simulink model "Complete_System_RatedVoltage"  (R2022b)
settings: Solver=VariableStepAuto  StartTime=0.0  StopTime=10  RelTol=1e-3
model workspace (MAT data in the model file):
  V_3phase = 121
libraries: spsDiodeLib x7, spsACVoltageSourceLib x3, spsMeanLib x2, spsSeriesRLCBranchLib x2, spsCurrentMeasurementLib x1, spsDCMachineLib x1, spsDCVoltageSourceLib x1, spsMosfetLib x1, spsVoltageMeasurementLib x1, spsPWMGeneratorDCDCLib x1, spsVariableRatioTransformerLib x1, sps_lib x1
settings Model: Creator=omers  LastModifiedBy=omers

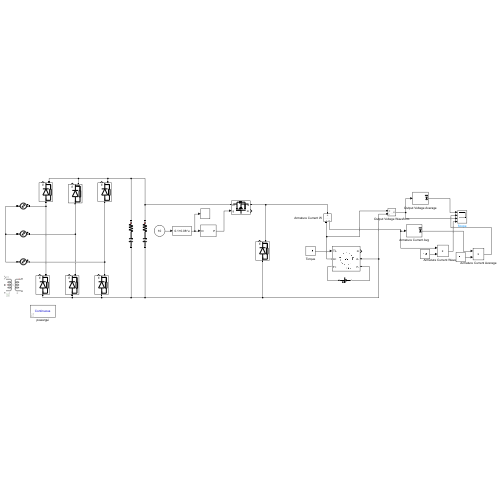
[thumbnail: Simulink's stored preview of the top-level diagram]
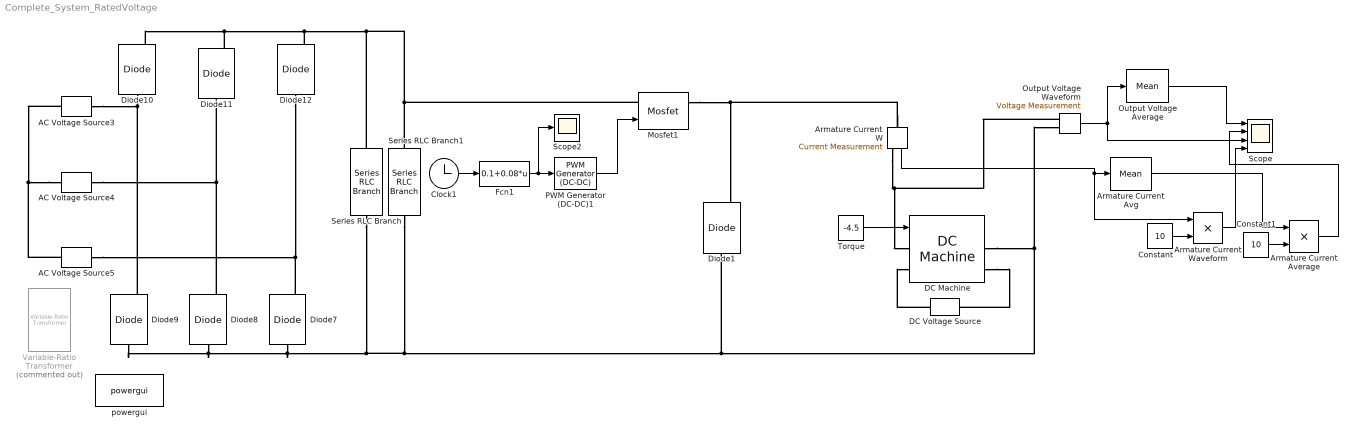
== system Complete_System_RatedVoltage ==
  AC Voltage Source3 : spsACVoltageSourceLib/AC Voltage Source  Amplitude=121  Phase=0  Frequency=50  SampleTime=0  Measurements=None  BusType=swing  Pref=10e3  Qref=0  Qmin=-inf  Qmax=+inf
  AC Voltage Source4 : spsACVoltageSourceLib/AC Voltage Source  Amplitude=121  Phase=-120  Frequency=50  SampleTime=0  Measurements=None  BusType=swing  Pref=10e3  Qref=0  Qmin=-inf  Qmax=+inf
  AC Voltage Source5 : spsACVoltageSourceLib/AC Voltage Source  Amplitude=121  Phase=-240  Frequency=50  SampleTime=0  Measurements=None  BusType=swing  Pref=10e3  Qref=0  Qmin=-inf  Qmax=+inf
  Armature Current Average : Product
  Armature Current Avg : spsMeanLib/Mean  Freq=50  Vinit=0  Ts=0
  Armature Current W : spsCurrentMeasurementLib/Current Measurement  PhasorSimulation=off  OutputType=Complex  PSBequivalent=0
  Armature Current Waveform : Product
  Clock1 : Clock
  Constant : Constant  Value=10
  Constant1 : Constant  Value=10
  DC Machine : spsDCMachineLib/DC Machine  PresetModel=No  MechanicalLoad=Torque TL  FieldType=Wound  ShowDetailedParameters=on  MeasurementBus=off  RLa="[ 0.8  0.0125]"  RLf="[ 210  23]"  Laf=1.8  MachineConstant=Torque constant (N.m/A)  Ke=1.8  Kt=1.8  J=1  Bm=0  Tf=0  w0=1  Ifinit=1.04761904756944  TsPowergui=0  TsBlock=-1
  DC Voltage Source : spsDCVoltageSourceLib/DC Voltage Source  Amplitude=220  Measurements=None
  Diode{1,7..12} (7 alike) : spsDiodeLib/Diode  Ron=0.001  Lon=0  Vf=0.8  IC=0  UseSnubber=0  Rs=500  Cs=250e-9  Measurements=on
  Fcn1 : Fcn  Expr=0.1+0.08*u
  Mosfet1 : spsMosfetLib/Mosfet  Ron=0.1  Lon=0  Rd=0.01  Vfd=0  IC=0  Rs=1e5  Cs=inf  Measurements=on
  Output Voltage Average : spsMeanLib/Mean  Freq=50  Vinit=0  Ts=0
  Output Voltage Waveform : spsVoltageMeasurementLib/Voltage Measurement  PhasorSimulation=off  OutputType=Complex  PSBequivalent=0
  PWM Generator (DC-DC)1 : spsPWMGeneratorDCDCLib/PWM Generator (DC-DC)  Fsw=1000  Ts=0
  Scope : Scope  NumInputPorts=4
  Scope2 : Scope
  Series RLC Branch : spsSeriesRLCBranchLib/Series RLC Branch  LConnTagsString=__new0  RConnTagsString=__new0  BranchType=RC  Resistance=0.0001  Inductance=1e-3  SetiL0=off  InitialCurrent=0  Capacitance=470e-6  Setx0=off  InitialVoltage=0  Measurements=None
  Series RLC Branch1 : spsSeriesRLCBranchLib/Series RLC Branch  LConnTagsString=__new0  RConnTagsString=__new0  BranchType=RC  Resistance=0.0001  Inductance=1e-3  SetiL0=off  InitialCurrent=0  Capacitance=470e-6  Setx0=off  InitialVoltage=0  Measurements=None
  Torque : Constant  Value=-4.5
  Variable-Ratio Transformer : spsVariableRatioTransformerLib/Variable-Ratio Transformer  Commented=on
      settings: LibrarySourceBlock=|
      | sps_lib/Passives/Variable-Ratio
      | Transformer
  powergui : sps_lib/powergui  Priority=1  SimulationMode=Continuous  SampleTime=50e-6  frequency=60  Iterations=50  frequencyindice=0  Pbase=100e6  ErrMax=1e-4  UnitsV=kV  UnitsW=MW  buscounter=0  FunctionMessages=off  echomessages=off  EnableUseOfTLC=off  CurrentSourceSwitches=off  DisableSnubberDevices=off  DisableRonSwitches=off  DisableVfSwitches=off  DisplayEquations=off  AutomaticDiscreteSolvers=off  SolverType=Tustin/Backward Euler (TBE)  Interpol=off  ExternalGateDelay=off  methode=off  Ts=100  x0status=blocks  SPID=on  SwTol=0  HookPort=off  NonlinearTolerance=1e-4  nMaxIteration=100  ContinueOnMaxIteration=off  RestoreLinks=warning  ResistiveCurrentMeasurement=off  Frange=[0:2:500]  Ylog=off  Xlog=on  ShowGrid=off  save=off  variable=ZData  structure=0  ZoomFFT=off  StartTime=0.0  cycles=1  DisplayStyle=1  fundamental=60  FreqAxis=off  MaxFrequency=1000  frequencyindicesteady=1  RmsSteady=1  display=off
  wires:
  Armature Current W/1 -> Armature Current Waveform/1, Armature Current Avg/1
  PWM Generator (DC-DC)1/1 -> Mosfet1/1
  Clock1/1 -> Fcn1/1
  Fcn1/1 -> PWM Generator (DC-DC)1/1, Scope2/1
  Output Voltage Average/1 -> Scope/1
  Torque/1 -> DC Machine/1
  Output Voltage Waveform/1 -> Output Voltage Average/1, Scope/3
  Constant/1 -> Armature Current Waveform/2
  Armature Current Waveform/1 -> Scope/4
  Armature Current Average/1 -> Scope/2
  Constant1/1 -> Armature Current Average/2
  Armature Current Avg/1 -> Armature Current Average/1
  connections:
  Armature Current W/RConn1 -- Output Voltage Waveform/LConn1 -- DC Machine/LConn1
  Diode8/LConn1 -- Diode7/LConn1 -- DC Machine/RConn1 -- Output Voltage Waveform/LConn2 -- Diode1/LConn1 -- Series RLC Branch1/RConn1 -- Series RLC Branch/RConn1 -- Diode9/LConn1
  DC Voltage Source/RConn1 -- DC Machine/LConn2
  DC Machine/RConn2 -- DC Voltage Source/LConn1
  Diode10/RConn1 -- Diode12/RConn1 -- Mosfet1/LConn1 -- Series RLC Branch1/LConn1 -- Series RLC Branch/LConn1 -- Diode11/RConn1
  Diode7/RConn1 -- AC Voltage Source5/RConn1 -- Diode12/LConn1
  Diode8/RConn1 -- Diode11/LConn1 -- AC Voltage Source4/RConn1
  AC Voltage Source4/LConn1 -- AC Voltage Source3/LConn1 -- AC Voltage Source5/LConn1
  Diode9/RConn1 -- AC Voltage Source3/RConn1 -- Diode10/LConn1
  Mosfet1/RConn1 -- Armature Current W/LConn1 -- Diode1/RConn1
